simulink model "furuta_sim_KL"  (R2020b)
settings: Solver=VariableStepAuto  StartTime=0.0  StopTime=5  MaxStep=1e-3  RelTol=1e-3
values from neighbouring files (symbols this model uses):
  A = A1    [furuta_script.m]    (also in practica2.m = [0 1; -2 -3])
  B = B1    [furuta_script.m]    (also in practica2.m = [10; 20])
  b1 = 1.00e-4    (= 0.0001)    [parameters.m]
  b2 = 2.80e-4    (= 0.00028)    [parameters.m]
  C = [1 0 0 0 0; 0 1 0 0 0]    [parameters.m]    (also in practica2.m = [1 0])
  CI = [-5*pi/180 -pi*5/180 0 0 0]    [furuta_script.m]
  g = 9.81    [parameters.m]
  J_hat_0 = J_hat_1+m2*L1^2    (= 0.0373463)    [parameters.m]
  J_hat_2 = J2+m2*l2^2    (= 0.0055028)    [parameters.m]
  Ki = -Ka(end)    [test_delete.m]
  Km = 0.090    (= 0.09)    [parameters.m]
  L = 0.005    [parameters.m]    (also in practica2_2.m = acker(Pss.A', Pss.c', Pdl)'; test_delete.m = acker(A',C',po)')
  L1 = 0.278    [parameters.m]
  l2 = 0.148    [parameters.m]
  m2 = 0.075    [parameters.m]
  n = length(A1)    [parameters.m]
  p = width(B1)    [parameters.m]    (also in test_delete.m = roots(conv([1 2*z*wn wn^2], [ 1 alpha*wn])))
  q = height(C)    [parameters.m]
  R = 7.80    (= 7.8)    [parameters.m]
undefined symbols (not defined in the file or in its folder): Abo, Ao, CIL, Lb, Lo, Nbari
settings Model: Creator=jorgegonzales  LastModifiedBy=jorgegonzales

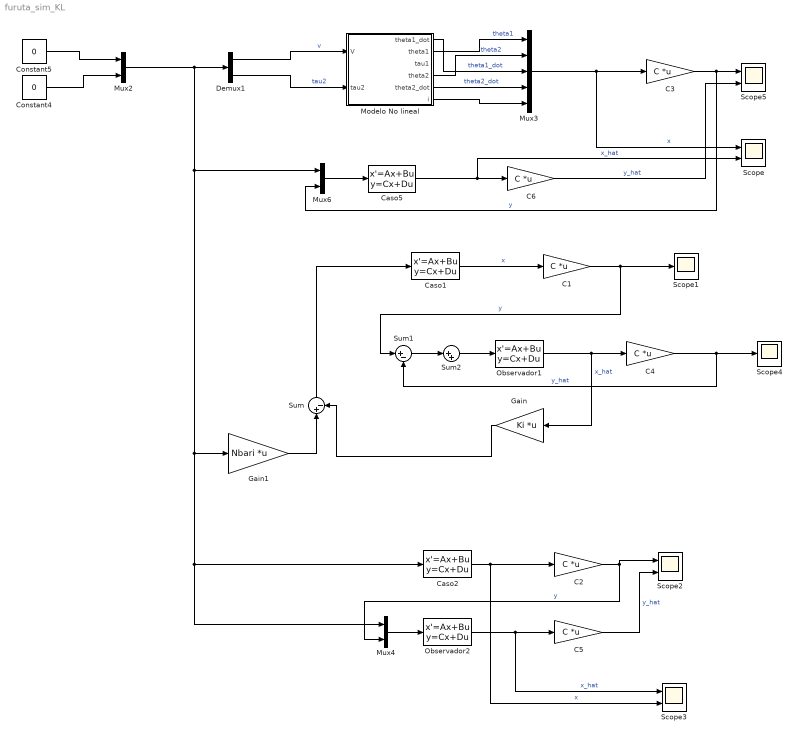
== system furuta_sim_KL ==
  C{1..6} (6 alike) : Gain  Gain=C  Multiplication=Matrix(K*u) (u vector)
  Caso1 : StateSpace  A=A  B=B  C=eye(n)  D=zeros(n,p)  InitialCondition=CI
  Caso2 : StateSpace  A=A  B=B  C=eye(n)  D=zeros(n,p)  InitialCondition=CI
  Caso5 : StateSpace  A=Ao  B=[B Lo]  C=eye(n)  D=zeros(n,p+q)  InitialCondition=CIL
  Constant4 : Constant  Value=0
  Constant5 : Constant  Value=0
  Demux1 : Demux  Outputs=2
  Gain : Gain  Gain=Ki  Multiplication=Matrix(K*u) (u vector)
  Gain1 : Gain  Gain=Nbari  Multiplication=Matrix(K*u) (u vector)
  Modelo No lineal : Subsystem
  Mux2 : Mux  Inputs=2
  Mux3 : Mux  Inputs=5
  Mux4 : Mux  Inputs=2
  Mux6 : Mux  Inputs=2
  Observador1 : StateSpace  A=A  B=B  C=eye(n)  D=zeros(n,p)  InitialCondition=CIL
  Observador2 : StateSpace  A=Abo  B=[B Lb]  C=eye(n)  D=zeros(n,p+q)  InitialCondition=CIL
  Scope{,2..3,5} (4 alike) : Scope  NumInputPorts=2
  Scope1 : Scope
  Scope4 : Scope
  Sum : Sum  Inputs=|+-
  Sum1 : Sum  Inputs=|+-
  Sum2 : Sum  Inputs=|++
  wires:
  C1/1 -> Sum1/1, Scope1/1  "y"
  Caso1/1 -> C1/1  "x"
  Modelo No lineal/2(theta1) -> Mux3/1  "theta1"
  Modelo No lineal/4(theta2) -> Mux3/2  "theta2"
  Modelo No lineal/1(theta1_dot) -> Mux3/3  "theta1_dot"
  Modelo No lineal/5(theta2_dot) -> Mux3/4  "theta2_dot"
  Modelo No lineal/6(i) -> Mux3/5
  Mux3/1 -> C3/1, Scope/1  "x"
  C3/1 -> Mux6/2, Scope5/1  "y"
  Observador1/1 -> Gain/1, C4/1  "x_hat"
  C5/1 -> Scope2/2  "y_hat"
  C2/1 -> Mux4/2, Scope2/1  "y"
  Caso2/1 -> Scope3/2, C2/1  "x"
  Observador2/1 -> Scope3/1, C5/1  "x_hat"
  Mux4/1 -> Observador2/1
  Constant5/1 -> Mux2/1
  Constant4/1 -> Mux2/2
  Mux2/1 -> Caso2/1, Mux4/1, Gain1/1, Mux6/1, Demux1/1
  Demux1/1 -> Modelo No lineal/1(V)  "v"
  Demux1/2 -> Modelo No lineal/2(tau2)  "tau2"
  Mux6/1 -> Caso5/1
  Caso5/1 -> Scope/2, C6/1  "x_hat"
  C6/1 -> Scope5/2  "y_hat"
  C4/1 -> Scope4/1, Sum1/2  "y_hat"
  Gain/1 -> Sum/2
  Sum/1 -> Caso1/1
  Gain1/1 -> Sum/1
  Sum1/1 -> Sum2/1
  Sum2/1 -> Observador1/1

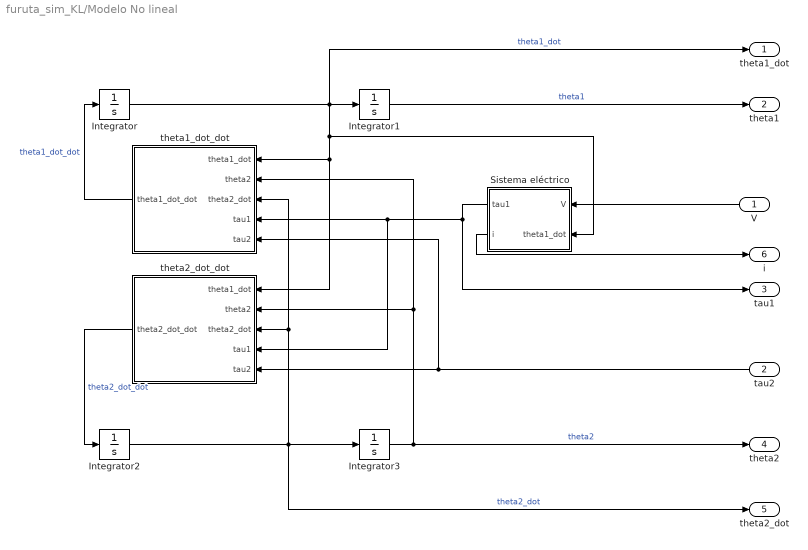
== system furuta_sim_KL/Modelo No lineal ==
  V : Inport
  tau2 : Inport  Port=2
  Integrator : Integrator  InitialCondition=CI(3)
  Integrator1 : Integrator  InitialCondition=CI(1)
  Integrator2 : Integrator  InitialCondition=CI(4)
  Integrator3 : Integrator  InitialCondition=CI(2)
  Sistema eléctrico : Subsystem
  theta1_dot_dot : Subsystem
  theta2_dot_dot : Subsystem
  theta1_dot : Outport
  theta1 : Outport  Port=2
  tau1 : Outport  Port=3
  theta2 : Outport  Port=4
  theta2_dot : Outport  Port=5
  i : Outport  Port=6
  wires:
  Sistema eléctrico/1(tau1) -> tau1/1, theta2_dot_dot/4(tau1), theta1_dot_dot/4(tau1)
  theta1_dot_dot/1(theta1_dot_dot) -> Integrator/1  "theta1_dot_dot"
  V/1 -> Sistema eléctrico/1(V)
  Integrator3/1 -> theta2/1, theta2_dot_dot/2(theta2), theta1_dot_dot/2(theta2)  "theta2"
  tau2/1 -> theta1_dot_dot/5(tau2), theta2_dot_dot/5(tau2)
  theta2_dot_dot/1(theta2_dot_dot) -> Integrator2/1  "theta2_dot_dot"
  Integrator1/1 -> theta1/1  "theta1"
  Integrator2/1 -> theta2_dot/1, theta2_dot_dot/3(theta2_dot), theta1_dot_dot/3(theta2_dot), Integrator3/1  "theta2_dot"
  Integrator/1 -> theta1_dot/1, Sistema eléctrico/2(theta1_dot), theta1_dot_dot/1(theta1_dot), theta2_dot_dot/1(theta1_dot), Integrator1/1  "theta1_dot"
  Sistema eléctrico/2(i) -> i/1

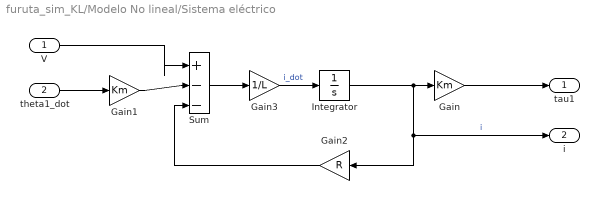
== system furuta_sim_KL/Modelo No lineal/Sistema eléctrico ==
  V : Inport
  theta1_dot : Inport  Port=2
  Gain : Gain  Gain=Km
  Gain1 : Gain  Gain=Km
  Gain2 : Gain  Gain=R
  Gain3 : Gain  Gain=1/L
  Integrator : Integrator  InitialCondition=CI(5)
  Sum : Sum  Inputs=|+--
  tau1 : Outport
  i : Outport  Port=2
  wires:
  Integrator/1 -> i/1, Gain2/1, Gain/1  "i"
  Gain/1 -> tau1/1
  theta1_dot/1 -> Gain1/1
  Gain1/1 -> Sum/2
  V/1 -> Sum/1
  Gain2/1 -> Sum/3
  Gain3/1 -> Integrator/1  "i_dot"
  Sum/1 -> Gain3/1

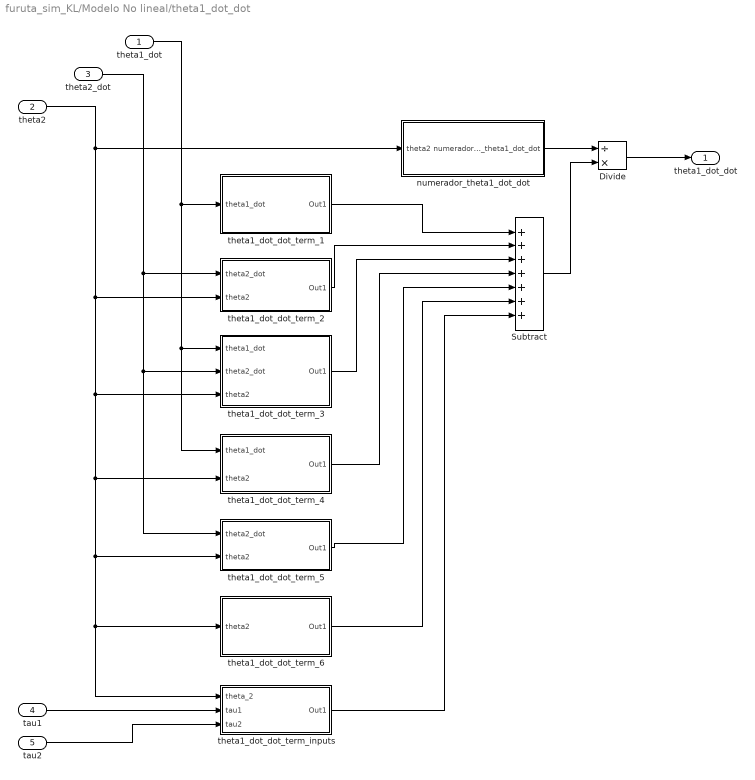
== system furuta_sim_KL/Modelo No lineal/theta1_dot_dot ==
  theta1_dot : Inport
  theta2 : Inport  Port=2
  theta2_dot : Inport  Port=3
  tau1 : Inport  Port=4
  tau2 : Inport  Port=5
  Divide : Product  Inputs=/*
  Subtract : Sum  Inputs=+++++++
  numerador_theta1_dot_dot : Subsystem
  theta1_dot_dot_term_1 : Subsystem
  theta1_dot_dot_term_2 : Subsystem
  theta1_dot_dot_term_3 : Subsystem
  theta1_dot_dot_term_4 : Subsystem
  theta1_dot_dot_term_5 : Subsystem
  theta1_dot_dot_term_6 : Subsystem
  theta1_dot_dot_term_inputs : Subsystem
  theta1_dot_dot : Outport
  wires:
  theta1_dot_dot_term_4/1(Out1) -> Subtract/4
  theta1_dot/1 -> theta1_dot_dot_term_3/1(theta1_dot), theta1_dot_dot_term_4/1(theta1_dot), theta1_dot_dot_term_1/1(theta1_dot)
  theta1_dot_dot_term_3/1(Out1) -> Subtract/3
  theta1_dot_dot_term_5/1(Out1) -> Subtract/5
  theta1_dot_dot_term_2/1(Out1) -> Subtract/2
  theta1_dot_dot_term_1/1(Out1) -> Subtract/1
  theta2_dot/1 -> theta1_dot_dot_term_5/1(theta2_dot), theta1_dot_dot_term_3/2(theta2_dot), theta1_dot_dot_term_2/1(theta2_dot)
  theta2/1 -> numerador_theta1_dot_dot/1(theta2), theta1_dot_dot_term_4/2(theta2), theta1_dot_dot_term_6/1(theta2), theta1_dot_dot_term_inputs/1(theta_2), theta1_dot_dot_term_5/2(theta2), theta1_dot_dot_term_3/3(theta2), theta1_dot_dot_term_2/2(theta2)
  tau1/1 -> theta1_dot_dot_term_inputs/2(tau1)
  tau2/1 -> theta1_dot_dot_term_inputs/3(tau2)
  theta1_dot_dot_term_6/1(Out1) -> Subtract/6
  theta1_dot_dot_term_inputs/1(Out1) -> Subtract/7
  numerador_theta1_dot_dot/1(numerador_theta1_dot_dot) -> Divide/1
  Subtract/1 -> Divide/2
  Divide/1 -> theta1_dot_dot/1

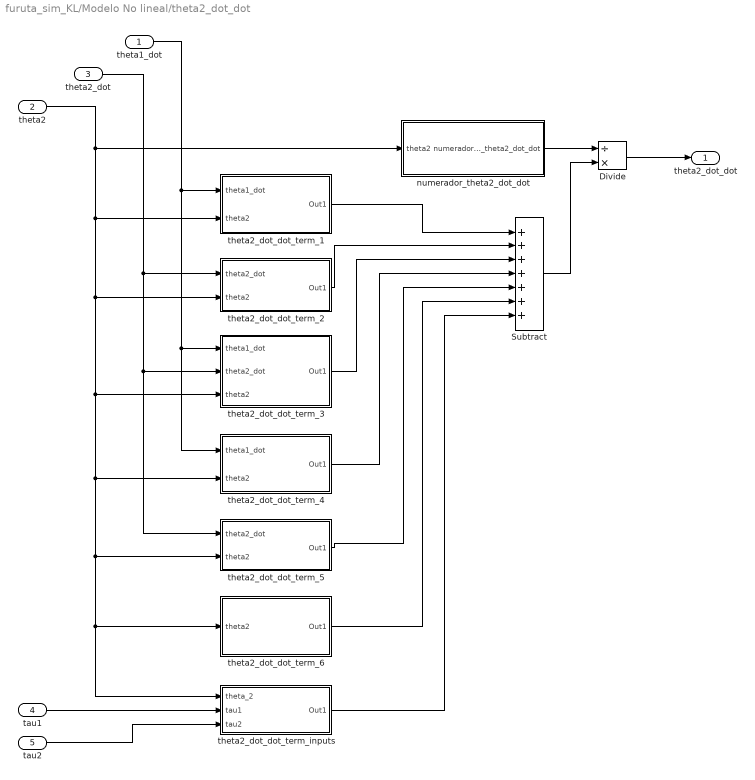
== system furuta_sim_KL/Modelo No lineal/theta2_dot_dot ==
  theta1_dot : Inport
  theta2 : Inport  Port=2
  theta2_dot : Inport  Port=3
  tau1 : Inport  Port=4
  tau2 : Inport  Port=5
  Divide : Product  Inputs=/*
  Subtract : Sum  Inputs=+++++++
  numerador_theta2_dot_dot : Subsystem
  theta2_dot_dot_term_1 : Subsystem
  theta2_dot_dot_term_2 : Subsystem
  theta2_dot_dot_term_3 : Subsystem
  theta2_dot_dot_term_4 : Subsystem
  theta2_dot_dot_term_5 : Subsystem
  theta2_dot_dot_term_6 : Subsystem
  theta2_dot_dot_term_inputs : Subsystem
  theta2_dot_dot : Outport
  wires:
  Divide/1 -> theta2_dot_dot/1
  Subtract/1 -> Divide/2
  numerador_theta2_dot_dot/1(numerador_theta2_dot_dot) -> Divide/1
  theta2_dot_dot_term_inputs/1(Out1) -> Subtract/7
  theta2_dot_dot_term_6/1(Out1) -> Subtract/6
  tau2/1 -> theta2_dot_dot_term_inputs/3(tau2)
  tau1/1 -> theta2_dot_dot_term_inputs/2(tau1)
  theta2/1 -> theta2_dot_dot_term_1/2(theta2), theta2_dot_dot_term_2/2(theta2), theta2_dot_dot_term_3/3(theta2), theta2_dot_dot_term_5/2(theta2), theta2_dot_dot_term_inputs/1(theta_2), theta2_dot_dot_term_6/1(theta2), theta2_dot_dot_term_4/2(theta2), numerador_theta2_dot_dot/1(theta2)
  theta2_dot/1 -> theta2_dot_dot_term_2/1(theta2_dot), theta2_dot_dot_term_3/2(theta2_dot), theta2_dot_dot_term_5/1(theta2_dot)
  theta2_dot_dot_term_1/1(Out1) -> Subtract/1
  theta2_dot_dot_term_2/1(Out1) -> Subtract/2
  theta2_dot_dot_term_5/1(Out1) -> Subtract/5
  theta2_dot_dot_term_3/1(Out1) -> Subtract/3
  theta1_dot/1 -> theta2_dot_dot_term_4/1(theta1_dot), theta2_dot_dot_term_3/1(theta1_dot), theta2_dot_dot_term_1/1(theta1_dot)
  theta2_dot_dot_term_4/1(Out1) -> Subtract/4

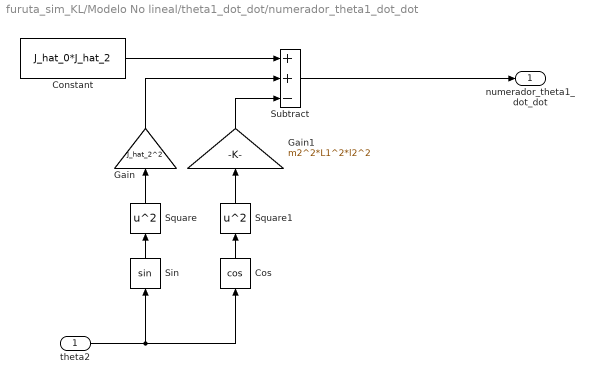
== system furuta_sim_KL/Modelo No lineal/theta1_dot_dot/numerador_theta1_dot_dot ==
  theta2 : Inport
  Constant : Constant  Value=J_hat_0*J_hat_2
  Cos : Trigonometry  Operator=cos
  Gain : Gain  Gain=J_hat_2^2
  Gain1 : Gain  Gain=m2^2*L1^2*l2^2
  Sin : Trigonometry
  Square : Math  Operator=square  SaturateOnIntegerOverflow=on
  Square1 : Math  Operator=square  SaturateOnIntegerOverflow=on
  Subtract : Sum  Inputs=++-
  numerador_theta1_dot_dot : Outport
  wires:
  Subtract/1 -> numerador_theta1_dot_dot/1
  Gain1/1 -> Subtract/3
  Sin/1 -> Square/1
  Gain/1 -> Subtract/2
  Constant/1 -> Subtract/1
  theta2/1 -> Cos/1, Sin/1
  Cos/1 -> Square1/1
  Square/1 -> Gain/1
  Square1/1 -> Gain1/1

== system furuta_sim_KL/Modelo No lineal/theta1_dot_dot/theta1_dot_dot_term_1 ==
  theta1_dot : Inport
  Gain2 : Gain  Gain=-1*J_hat_2*b1
  Out1 : Outport
  wires:
  theta1_dot/1 -> Gain2/1
  Gain2/1 -> Out1/1

== system furuta_sim_KL/Modelo No lineal/theta1_dot_dot/theta1_dot_dot_term_2 ==
  theta2_dot : Inport
  theta2 : Inport  Port=2
  Cos1 : Trigonometry  Operator=cos
  Divide1 : Product  Inputs=**
  Gain3 : Gain  Gain=m2*L1*l2*b2
  Out1 : Outport
  wires:
  Gain3/1 -> Divide1/1
  theta2_dot/1 -> Divide1/2
  Cos1/1 -> Gain3/1
  theta2/1 -> Cos1/1
  Divide1/1 -> Out1/1

== system furuta_sim_KL/Modelo No lineal/theta1_dot_dot/theta1_dot_dot_term_3 ==
  theta1_dot : Inport
  theta2_dot : Inport  Port=2
  theta2 : Inport  Port=3
  Divide2 : Product  Inputs=***
  Gain4 : Gain  Gain=2
  Gain5 : Gain  Gain=-1*J_hat_2^2
  Sin1 : Trigonometry
  Out1 : Outport
  wires:
  theta2_dot/1 -> Divide2/3
  Sin1/1 -> Gain5/1
  theta1_dot/1 -> Divide2/2
  Divide2/1 -> Out1/1
  theta2/1 -> Gain4/1
  Gain4/1 -> Sin1/1
  Gain5/1 -> Divide2/1

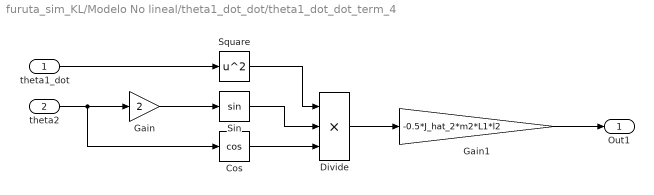
== system furuta_sim_KL/Modelo No lineal/theta1_dot_dot/theta1_dot_dot_term_4 ==
  theta1_dot : Inport
  theta2 : Inport  Port=2
  Cos : Trigonometry  Operator=cos
  Divide : Product  Inputs=***
  Gain : Gain  Gain=2
  Gain1 : Gain  Gain=-0.5*J_hat_2*m2*L1*l2
  Sin : Trigonometry
  Square : Math  Operator=square  SaturateOnIntegerOverflow=on
  Out1 : Outport
  wires:
  Gain/1 -> Sin/1
  Divide/1 -> Gain1/1
  theta1_dot/1 -> Square/1
  Square/1 -> Divide/1
  Sin/1 -> Divide/2
  theta2/1 -> Cos/1, Gain/1
  Cos/1 -> Divide/3
  Gain1/1 -> Out1/1

== system furuta_sim_KL/Modelo No lineal/theta1_dot_dot/theta1_dot_dot_term_5 ==
  theta2_dot : Inport
  theta2 : Inport  Port=2
  Divide : Product  Inputs=**
  Gain : Gain  Gain=J_hat_2*m2*L1*l2
  Sin : Trigonometry
  Square : Math  Operator=square  SaturateOnIntegerOverflow=on
  Out1 : Outport
  wires:
  theta2_dot/1 -> Square/1
  Square/1 -> Divide/2
  Sin/1 -> Divide/1
  Divide/1 -> Gain/1
  theta2/1 -> Sin/1
  Gain/1 -> Out1/1

== system furuta_sim_KL/Modelo No lineal/theta1_dot_dot/theta1_dot_dot_term_6 ==
  theta2 : Inport
  Gain : Gain  Gain=2
  Gain1 : Gain  Gain=0.5*m2^2*l2^2*L1*g
  Sin : Trigonometry
  Out1 : Outport
  wires:
  theta2/1 -> Gain/1
  Gain1/1 -> Out1/1
  Gain/1 -> Sin/1
  Sin/1 -> Gain1/1

== system furuta_sim_KL/Modelo No lineal/theta1_dot_dot/theta1_dot_dot_term_inputs ==
  theta_2 : Inport
  tau1 : Inport  Port=2
  tau2 : Inport  Port=3
  Cos : Trigonometry  Operator=cos
  Divide : Product  Inputs=**
  Gain : Gain  Gain=J_hat_2
  Gain1 : Gain  Gain=-1*m2*L1*l2
  Sum : Sum  Inputs=|++
  Out1 : Outport
  wires:
  theta_2/1 -> Cos/1
  Sum/1 -> Out1/1
  Gain/1 -> Sum/1
  Cos/1 -> Divide/2
  tau1/1 -> Gain/1
  tau2/1 -> Divide/1
  Gain1/1 -> Sum/2
  Divide/1 -> Gain1/1

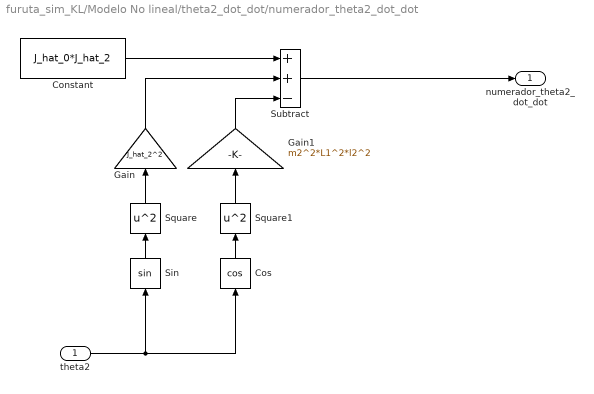
== system furuta_sim_KL/Modelo No lineal/theta2_dot_dot/numerador_theta2_dot_dot ==
  theta2 : Inport
  Constant : Constant  Value=J_hat_0*J_hat_2
  Cos : Trigonometry  Operator=cos
  Gain : Gain  Gain=J_hat_2^2
  Gain1 : Gain  Gain=m2^2*L1^2*l2^2
  Sin : Trigonometry
  Square : Math  Operator=square  SaturateOnIntegerOverflow=on
  Square1 : Math  Operator=square  SaturateOnIntegerOverflow=on
  Subtract : Sum  Inputs=++-
  numerador_theta2_dot_dot : Outport
  wires:
  Square1/1 -> Gain1/1
  Square/1 -> Gain/1
  Cos/1 -> Square1/1
  theta2/1 -> Cos/1, Sin/1
  Constant/1 -> Subtract/1
  Gain/1 -> Subtract/2
  Sin/1 -> Square/1
  Gain1/1 -> Subtract/3
  Subtract/1 -> numerador_theta2_dot_dot/1

== system furuta_sim_KL/Modelo No lineal/theta2_dot_dot/theta2_dot_dot_term_1 ==
  theta1_dot : Inport
  theta2 : Inport  Port=2
  Cos : Trigonometry  Operator=cos
  Divide : Product  Inputs=**
  Gain2 : Gain  Gain=m2*L1*l2*b1
  Out1 : Outport
  wires:
  Gain2/1 -> Out1/1
  theta2/1 -> Cos/1
  Cos/1 -> Divide/2
  theta1_dot/1 -> Divide/1
  Divide/1 -> Gain2/1

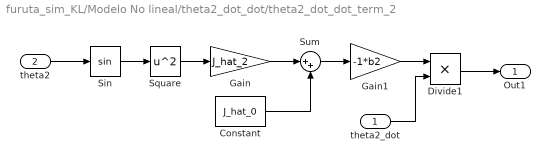
== system furuta_sim_KL/Modelo No lineal/theta2_dot_dot/theta2_dot_dot_term_2 ==
  theta2_dot : Inport
  theta2 : Inport  Port=2
  Constant : Constant  Value=J_hat_0
  Divide1 : Product  Inputs=**
  Gain : Gain  Gain=J_hat_2
  Gain1 : Gain  Gain=-1*b2
  Sin : Trigonometry
  Square : Math  Operator=square  SaturateOnIntegerOverflow=on
  Sum : Sum  Inputs=|++
  Out1 : Outport
  wires:
  Divide1/1 -> Out1/1
  theta2/1 -> Sin/1
  Sin/1 -> Square/1
  Square/1 -> Gain/1
  Gain/1 -> Sum/1
  Constant/1 -> Sum/2
  Sum/1 -> Gain1/1
  Gain1/1 -> Divide1/1
  theta2_dot/1 -> Divide1/2

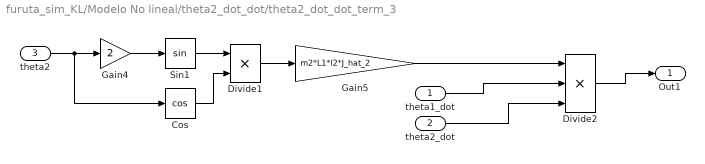
== system furuta_sim_KL/Modelo No lineal/theta2_dot_dot/theta2_dot_dot_term_3 ==
  theta1_dot : Inport
  theta2_dot : Inport  Port=2
  theta2 : Inport  Port=3
  Cos : Trigonometry  Operator=cos
  Divide1 : Product  Inputs=**
  Divide2 : Product  Inputs=***
  Gain4 : Gain  Gain=2
  Gain5 : Gain  Gain=m2*L1*l2*J_hat_2
  Sin1 : Trigonometry
  Out1 : Outport
  wires:
  Gain5/1 -> Divide2/1
  Gain4/1 -> Sin1/1
  theta2/1 -> Cos/1, Gain4/1
  Divide2/1 -> Out1/1
  theta1_dot/1 -> Divide2/2
  theta2_dot/1 -> Divide2/3
  Sin1/1 -> Divide1/1
  Cos/1 -> Divide1/2
  Divide1/1 -> Gain5/1

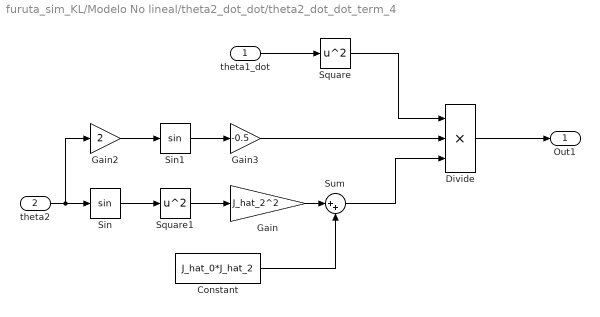
== system furuta_sim_KL/Modelo No lineal/theta2_dot_dot/theta2_dot_dot_term_4 ==
  theta1_dot : Inport
  theta2 : Inport  Port=2
  Constant : Constant  Value=J_hat_0*J_hat_2
  Divide : Product  Inputs=***
  Gain : Gain  Gain=J_hat_2^2
  Gain2 : Gain  Gain=2
  Gain3 : Gain  Gain=-0.5
  Sin : Trigonometry
  Sin1 : Trigonometry
  Square : Math  Operator=square  SaturateOnIntegerOverflow=on
  Square1 : Math  Operator=square  SaturateOnIntegerOverflow=on
  Sum : Sum  Inputs=|++
  Out1 : Outport
  wires:
  Divide/1 -> Out1/1
  Square/1 -> Divide/1
  theta1_dot/1 -> Square/1
  theta2/1 -> Gain2/1, Sin/1
  Sin/1 -> Square1/1
  Square1/1 -> Gain/1
  Gain/1 -> Sum/1
  Constant/1 -> Sum/2
  Gain2/1 -> Sin1/1
  Sin1/1 -> Gain3/1
  Gain3/1 -> Divide/2
  Sum/1 -> Divide/3

== system furuta_sim_KL/Modelo No lineal/theta2_dot_dot/theta2_dot_dot_term_5 ==
  theta2_dot : Inport
  theta2 : Inport  Port=2
  Divide : Product  Inputs=**
  Gain : Gain  Gain=-0.5*m2^2*L1^2*l2^2
  Gain1 : Gain  Gain=2
  Sin : Trigonometry
  Square : Math  Operator=square  SaturateOnIntegerOverflow=on
  Out1 : Outport
  wires:
  Gain/1 -> Out1/1
  Divide/1 -> Gain/1
  Sin/1 -> Divide/1
  Square/1 -> Divide/2
  theta2_dot/1 -> Square/1
  theta2/1 -> Gain1/1
  Gain1/1 -> Sin/1

== system furuta_sim_KL/Modelo No lineal/theta2_dot_dot/theta2_dot_dot_term_6 ==
  theta2 : Inport
  Constant : Constant  Value=J_hat_0
  Divide : Product  Inputs=**
  Gain : Gain  Gain=J_hat_2
  Gain1 : Gain  Gain=-1*m2*l2*g
  Sin : Trigonometry
  Square : Math  Operator=square  SaturateOnIntegerOverflow=on
  Sum : Sum  Inputs=|++
  Out1 : Outport
  wires:
  Gain1/1 -> Out1/1
  theta2/1 -> Sin/1
  Sin/1 -> Divide/1, Square/1
  Square/1 -> Gain/1
  Gain/1 -> Sum/1
  Constant/1 -> Sum/2
  Sum/1 -> Divide/2
  Divide/1 -> Gain1/1

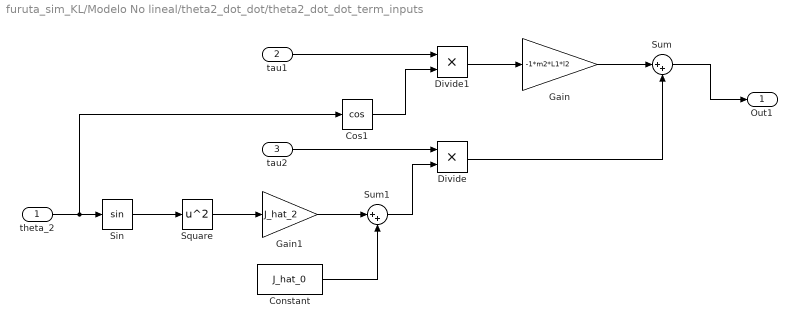
== system furuta_sim_KL/Modelo No lineal/theta2_dot_dot/theta2_dot_dot_term_inputs ==
  theta_2 : Inport
  tau1 : Inport  Port=2
  tau2 : Inport  Port=3
  Constant : Constant  Value=J_hat_0
  Cos1 : Trigonometry  Operator=cos
  Divide : Product  Inputs=**
  Divide1 : Product  Inputs=**
  Gain : Gain  Gain=-1*m2*L1*l2
  Gain1 : Gain  Gain=J_hat_2
  Sin : Trigonometry
  Square : Math  Operator=square  SaturateOnIntegerOverflow=on
  Sum : Sum  Inputs=|++
  Sum1 : Sum  Inputs=|++
  Out1 : Outport
  wires:
  Divide/1 -> Sum/2
  tau2/1 -> Divide/1
  Sum/1 -> Out1/1
  tau1/1 -> Divide1/1
  Cos1/1 -> Divide1/2
  Gain/1 -> Sum/1
  Divide1/1 -> Gain/1
  theta_2/1 -> Cos1/1, Sin/1
  Sin/1 -> Square/1
  Square/1 -> Gain1/1
  Gain1/1 -> Sum1/1
  Constant/1 -> Sum1/2
  Sum1/1 -> Divide/2
